simulink model "Lure_model_gradient_simulation"  (R2017b)
settings: Solver=VariableStepAuto  StartTime=0.0  StopTime=P*T-T/n  MaxStep=1e-2  RelTol=nfi_pars.RelTol  AbsTol=nfi_pars.AbsTol
values from neighbouring files (symbols this model uses):
  n = mtf_pars.n    [MTF_Sensitivity.m]    (also in MTF_Solution.m; NFISim_Solution.m = nfi_pars.n; NFISim_Solution2.m = nfi_pars.n)
  T = mtf_pars.T    [MTF_Solution.m]    (also in NFISim_Solution.m = nfi_pars.T; NFISim_Solution2.m = nfi_pars.T)
undefined symbols (not defined in the file or in its folder): luresys
settings Model: Creator=s128538  LastModifiedBy=nverv

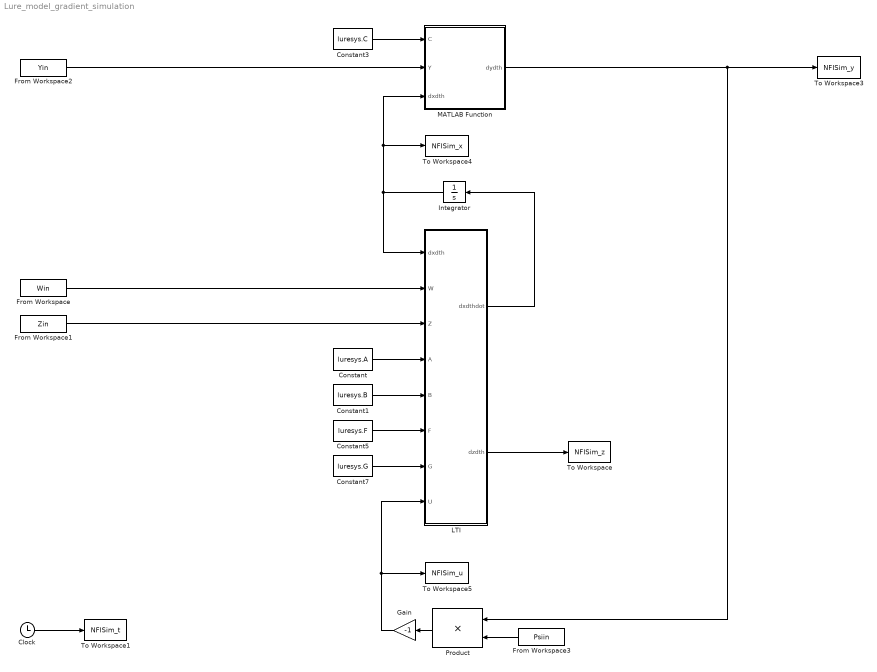
== system Lure_model_gradient_simulation ==
  Clock : Clock
  Constant : Constant  Value=luresys.A
  Constant1 : Constant  Value=luresys.B  VectorParams1D=off
  Constant3 : Constant  Value=luresys.C  VectorParams1D=off
  Constant5 : Constant  Value=luresys.F  VectorParams1D=off
  Constant7 : Constant  Value=luresys.G  VectorParams1D=off
  From Workspace : FromWorkspace  VariableName=Win
  From Workspace1 : FromWorkspace  VariableName=Zin
  From Workspace2 : FromWorkspace  VariableName=Yin
  From Workspace3 : FromWorkspace  VariableName=Psiin
  Gain : Gain  Gain=-1
  Integrator : Integrator  InitialCondition=[1;0;1.5;0]
  LTI : MATLAB Function  TreatAsAtomicUnit=on
  MATLAB Function : MATLAB Function  TreatAsAtomicUnit=on
  Product : Product
  To Workspace : ToWorkspace  VariableName=NFISim_z  SampleTime=T/n
  To Workspace1 : ToWorkspace  VariableName=NFISim_t  SampleTime=T/n
  To Workspace3 : ToWorkspace  VariableName=NFISim_y  SampleTime=T/n
  To Workspace4 : ToWorkspace  VariableName=NFISim_x  SampleTime=T/n
  To Workspace5 : ToWorkspace  VariableName=NFISim_u  SampleTime=T/n
  wires:
  LTI/1(dxdthdot) -> Integrator/1
  Integrator/1 -> LTI/1(dxdth), To Workspace4/1, MATLAB Function/3(dxdth)
  Product/1 -> Gain/1
  Constant/1 -> LTI/4(A)
  Constant1/1 -> LTI/5(B)
  Constant5/1 -> LTI/6(F)
  Constant7/1 -> LTI/7(G)
  From Workspace/1 -> LTI/2(W)
  LTI/2(dzdth) -> To Workspace/1
  MATLAB Function/1(dydth) -> To Workspace3/1, Product/1
  Clock/1 -> To Workspace1/1
  From Workspace1/1 -> LTI/3(Z)
  From Workspace3/1 -> Product/2
  From Workspace2/1 -> MATLAB Function/2(Y)
  Constant3/1 -> MATLAB Function/1(C)
  Gain/1 -> To Workspace5/1, LTI/8(U)

== matlab function Lure_model_gradient_simulation/MATLAB Function ==
  data: C input; Y input; dxdth input; dydth output
function dydth =  dydthfunc(C,Y,dxdth)

    dydth    = C*dxdth + Y;
end

== matlab function Lure_model_gradient_simulation/LTI ==
  data: dxdth input; W input; Z input; A input; B input; F input; G input; U input; dxdthdot output; dzdth output
function [dxdthdot,dzdth] = fcn(dxdth,W,Z,A,B,F,G, U)

dxdthdot = A*dxdth + B*U + W;
dzdth    = F*dxdth + G*U + Z;
